simulink model "BBB_GPIO_Read_Write_Test_LibraryBlock"  (R2013a)
settings: Solver=FixedStepDiscrete  StartTime=0.0  StopTime=inf  FixedStep=0.01  RelTol=1e-3
libraries: simulink x5, BLACKlink x2
settings Model: SimulationMode=external  ExtModeTrigDuration=100  Creator=rdustinkahawita  LastModifiedBy=rdustinkahawita
settings OptimizationCC: OptimizeModelRefInitCode=on  LifeSpan=1
settings DebuggingCC: SolverPrmCheckMsg=none  StrictBusMsg=Warning
settings HardwareCC: ProdLargestAtomicInteger=Long  ProdLargestAtomicFloat=Double  ProdEndianess=LittleEndian  ProdHWDeviceType=ARM Compatible->ARM Cortex
settings RTWCC: SystemTargetFile=realtime.tlc  GenerateMakefile=off  TemplateMakefile=realtime.tmf  Description=Run on Target Hardware  RTWVerbose=off  ProcessScript=realtime_make_rtw_hook
settings STFCustomTargetCC: TargetLibSuffix=.a  GenerateSampleERTMain=on  ERTCustomFileBanners=on  SupportNonInlinedSFcns=off  SupportVariableSizeSignals=on  MATLABClassNameForMDSCustomization=Simulink.SoftwareTarget.ERTCustomization  SystemTargetFile=realtime.tlc
settings ERTTargetCC: ParMdlRefBuildCompliant=off  CompOptLevelCompliant=off  ConcurrentExecutionCompliant=off  CombineOutputUpdateFcns=off  ERTFirstTimeCompliant=off  SupportContinuousTime=on  SupportVariableSizeSignals=on  ModelStepFunctionPrototypeControlCompliant=off  CPPClassGenCompliant=off  ExtMode=on  ExtModeMexArgs='192.168.7.2' 0 17725  ERTSrcFileBannerTemplate=realtime_code_template.cgt  ERTHdrFileBannerTemplate=realtime_code_template.cgt  ERTDataSrcFileTemplate=realtime_code_template.cgt  ERTDataHdrFileTemplate=realtime_code_template.cgt  ERTCustomFileTemplate=realtime_file_process.tlc

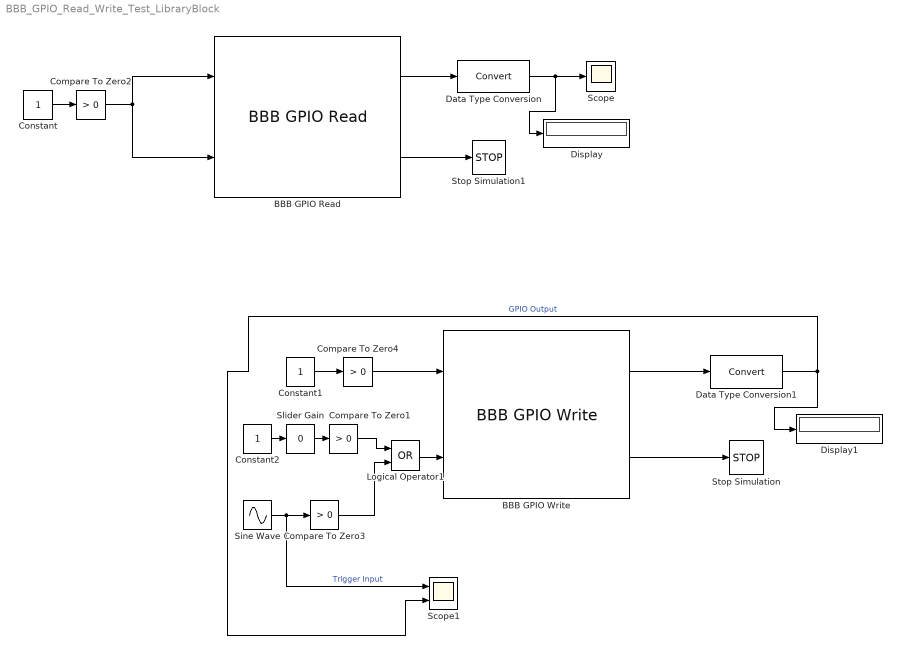
== system BBB_GPIO_Read_Write_Test_LibraryBlock ==
  BBB GPIO Read : BLACKlink/BBB GPIO Read  BBB_GPIOPin=Pin P9_23 -> GPIO[49]  BBB_DebugInfo=No Debug Info
  BBB GPIO Write : BLACKlink/BBB GPIO Write  BBB_GPIOPin=Pin P9_12 -> GPIO[60]  BBB_DebugInfo=Debug Level 0 - Basic Info Only
  Compare To Zero{1..4} (4 alike) : simulink/Logic and Bit Operations/Compare To Zero  relop=>  OutDataTypeStr=boolean
  Constant : Constant
  Constant1 : Constant
  Constant2 : Constant
  Data Type Conversion : DataTypeConversion
  Data Type Conversion1 : DataTypeConversion
  Display : Display
  Display1 : Display
  Logical Operator1 : Logic  Operator=OR  AllPortsSameDT=off  OutDataTypeStr=boolean
  Scope : Scope
      settings: TimeRange=30
  Scope1 : Scope  NumInputPorts=2
      settings: ShowLegends=on  YMin=-5~-5  YMax=5~5
  Sine Wave : Sin  Frequency=4
  Slider Gain : simulink/Math Operations/Slider Gain  low=0  gain=0  high=1
  Stop Simulation : Stop
  Stop Simulation1 : Stop
  wires:
  BBB GPIO Write/1 -> Data Type Conversion1/1
  BBB GPIO Read/1 -> Data Type Conversion/1
  Data Type Conversion/1 -> Display/1, Scope/1
  Data Type Conversion1/1 -> Scope1/2, Display1/1  "GPIO Output"
  BBB GPIO Write/2 -> Stop Simulation/1
  BBB GPIO Read/2 -> Stop Simulation1/1
  Compare To Zero2/1 -> BBB GPIO Read/2, BBB GPIO Read/1
  Slider Gain/1 -> Compare To Zero1/1
  Constant2/1 -> Slider Gain/1
  Logical Operator1/1 -> BBB GPIO Write/2
  Compare To Zero1/1 -> Logical Operator1/1
  Compare To Zero3/1 -> Logical Operator1/2
  Sine Wave/1 -> Scope1/1, Compare To Zero3/1  "Trigger Input"
  Constant/1 -> Compare To Zero2/1
  Constant1/1 -> Compare To Zero4/1
  Compare To Zero4/1 -> BBB GPIO Write/1
